simulink model "atrias_boom_nmSt_kinSw_v3"  (R2015a)
settings: Solver=ode23t  StartTime=0.0  StopTime=t_end  FixedStep=0.001  MaxStep=1e-3  RelTol=1e-3
InitFcn:
  | addpath('../common/')
  | colors
StartFcn:
  | tic
StopFcn:
  | %stopscript
values from neighbouring files (symbols this model uses):
  dt_a_dTrunk_boom = 5    [main_1_nmSt_kinSw.m]    (also in main_2_nmSt_kinSw_v2.m; main_3_nmSt_kinSw_v3.m; main_4_nmSt_kinSw_v4.m)
  dt_fade_boomCtrl = 2    [main_1_nmSt_kinSw.m]    (also in main_2_nmSt_kinSw_v2.m; main_3_nmSt_kinSw_v3.m; main_4_nmSt_kinSw_v4.m)
  initial_boom_yaw = 15*pi/180    (= 0.261799387799)    [main_2_nmSt_kinSw_v2.m]    (also in main_3_nmSt_kinSw_v3.m; main_4_nmSt_kinSw_v4.m)
  kd_boom_roll_Ctrl = 0    [main_1_nmSt_kinSw - Copy.m]    (also in main_1_nmSt_kinSw.m; main_2_nmSt_kinSw_v2.m; main_3_nmSt_kinSw_v3.m; main_4_nmSt_kinSw_v4.m)
  kd_boom_yaw_Ctrl = 0.1*kp_boom_yaw_Ctrl    (= 100000000)    [main_1_nmSt_kinSw - Copy.m]    (also in main_1_nmSt_kinSw.m = 1000000000; main_2_nmSt_kinSw_v2.m = 10000000; main_3_nmSt_kinSw_v3.m = 10000000; main_4_nmSt_kinSw_v4.m = 10000000)
  kd_motor = 0.90*2*sqrt(3.75*kp_motor)    [main_1_nmSt_kinSw - Copy.m]
  kinSw_alpha_start = 100*pi/180    (= 1.74532925199)    [main_1_nmSt_kinSw - Copy.m]    (also in main_1_nmSt_kinSw.m = 1.91986217719; main_2_nmSt_kinSw_v2.m = 1.83259571459; main_3_nmSt_kinSw_v3.m = 1.83259571459; main_4_nmSt_kinSw_v4.m = 1.83259571459)
  kinSw_alpha_tgt = 80*pi/180    (= 1.3962634016)    [main_1_nmSt_kinSw - Copy.m]    (also in main_1_nmSt_kinSw.m = 1.2217304764; main_2_nmSt_kinSw_v2.m = 1.2217304764; main_3_nmSt_kinSw_v3.m = 1.2217304764; main_4_nmSt_kinSw_v4.m = 1.2217304764)
  kinSw_t_start = 1.5    [main_1_nmSt_kinSw - Copy.m]    (also in main_1_nmSt_kinSw.m; main_2_nmSt_kinSw_v2.m = 0.5; main_3_nmSt_kinSw_v3.m = 0.5; main_4_nmSt_kinSw_v4.m = 0.5)
  kp_boom_roll_Ctrl = 0    [main_1_nmSt_kinSw - Copy.m]    (also in main_1_nmSt_kinSw.m; main_2_nmSt_kinSw_v2.m; main_3_nmSt_kinSw_v3.m; main_4_nmSt_kinSw_v4.m)
  kp_boom_yaw_Ctrl = 1e9    (= 1000000000)    [main_1_nmSt_kinSw - Copy.m]    (also in main_1_nmSt_kinSw.m = 10000000000; main_2_nmSt_kinSw_v2.m = 100000000; main_3_nmSt_kinSw_v3.m = 100000000; main_4_nmSt_kinSw_v4.m = 100000000)
  kp_motor = 3000    [main_1_nmSt_kinSw - Copy.m]
  max_back_bar_angle = 262.4*pi/180    (= 4.57974395723)    [main_1_nmSt_kinSw - Copy.m]
  max_front_bar_angle = 194.8*pi/180    (= 3.39990138288)    [main_1_nmSt_kinSw - Copy.m]
  min_back_bar_angle = 165.0*pi/180    (= 2.87979326579)    [main_1_nmSt_kinSw - Copy.m]
  min_front_bar_angle = 98.0*pi/180    (= 1.71042266695)    [main_1_nmSt_kinSw - Copy.m]
  poser_LLegAlp = (initial_l_leg_angle -pi/2)*180/pi    (= 105)    [main_2_nmSt_kinSw_v2.m]    (also in main_3_nmSt_kinSw_v3.m; main_4_nmSt_kinSw_v4.m)
  poser_LLegLen = initial_l_leg_length    (= 0.88)    [main_2_nmSt_kinSw_v2.m]    (also in main_3_nmSt_kinSw_v3.m; main_4_nmSt_kinSw_v4.m)
  poser_RLegAlp = (initial_r_leg_angle -pi/2)*180/pi    (= 75)    [main_2_nmSt_kinSw_v2.m]    (also in main_3_nmSt_kinSw_v3.m; main_4_nmSt_kinSw_v4.m)
  poser_RLegLen = initial_r_leg_length    (= 0.9)    [main_2_nmSt_kinSw_v2.m]    (also in main_3_nmSt_kinSw_v3.m; main_4_nmSt_kinSw_v4.m)
  tEnd_boomCtrl = t_end    (= 20)    [main_1_nmSt_kinSw - Copy.m]    (also in main_1_nmSt_kinSw.m = 3; main_2_nmSt_kinSw_v2.m = 7.5; main_3_nmSt_kinSw_v3.m = 7.5; main_4_nmSt_kinSw_v4.m = 7.5)
  tStart_boomCtrl = 1    [main_1_nmSt_kinSw - Copy.m]    (also in main_1_nmSt_kinSw.m = 0; main_2_nmSt_kinSw_v2.m = 0.5; main_3_nmSt_kinSw_v3.m = 0.5; main_4_nmSt_kinSw_v4.m = 0.5)
  tune_kinSw_alpha_start = kinSw_alpha_start*180/pi    (= 105)    [main_2_nmSt_kinSw_v2.m]    (also in main_3_nmSt_kinSw_v3.m; main_4_nmSt_kinSw_v4.m)
  tune_kinSw_alpha_tgt = kinSw_alpha_tgt*180/pi    (= 70)    [main_2_nmSt_kinSw_v2.m]    (also in main_3_nmSt_kinSw_v3.m; main_4_nmSt_kinSw_v4.m)
  tune_kinSw_len_min = kinSw_lclr    (= 0.7)    [main_2_nmSt_kinSw_v2.m]    (also in main_3_nmSt_kinSw_v3.m = 0.6)
  tune_kinSw_len_tgt = kinSw_len_tgt    (= 0.9)    [main_2_nmSt_kinSw_v2.m]    (also in main_3_nmSt_kinSw_v3.m)
  tune_M1_G = St_FGain_VAS*FmaxVAS    [main_2_nmSt_kinSw_v2.m]    (also in main_3_nmSt_kinSw_v3.m; main_4_nmSt_kinSw_v4.m)
  tune_M3_0 = CtrlPar_theta0*180/pi    [main_2_nmSt_kinSw_v2.m]    (also in main_3_nmSt_kinSw_v3.m; main_4_nmSt_kinSw_v4.m)
  tune_M3_D = St_GainDTh_HFL    [main_2_nmSt_kinSw_v2.m]    (also in main_3_nmSt_kinSw_v3.m; main_4_nmSt_kinSw_v4.m)
  tune_M3_P = St_GainTh_HFL    [main_2_nmSt_kinSw_v2.m]    (also in main_3_nmSt_kinSw_v3.m; main_4_nmSt_kinSw_v4.m)
  tune_M4_G = 1    [main_3_nmSt_kinSw_v3.m]    (also in main_4_nmSt_kinSw_v4.m)
  v_dTrunk_boom = 1.3    [main_1_nmSt_kinSw.m]    (also in main_2_nmSt_kinSw_v2.m; main_3_nmSt_kinSw_v3.m; main_4_nmSt_kinSw_v4.m)
undefined symbols (not defined in the file or in its folder): A1_notch_f1, A2_notch_f1, A_lpf_dtau, A_lpf_velocity, ankle_stiffness, B1_lpf_dtau, B1_lpf_velocity, B1_notch_f1, B2_lpf_dtau, B2_lpf_velocity, B2_notch_f1, b_hmotor, b_leg_spring, b_rotor, base_color_d, boom_color_d, boom_mount_to_center_diagonal, breakaway_friction, c_jointstop, contactThr, coulomb_friction, d_com, delta_phi_max, delta_phi_max_buffer, delta_phi_max_dropoff, delta_phi_min, fblink_color_d, floor_color_d, FmaxBFSH, FmaxGLU, FmaxHAM, FmaxHFL, FmaxRF, FmaxVAS, foot_color_d, FPCtrlPar, friction_linear_zone, g, gain_nodes_sea_torque, HIP_MTR_MAX_CONT_TORQUE, HIP_MTR_MAX_TORQUE, hshaft_color_d, initial_boom_pitch, initial_boom_roll, initial_hip_roll, initial_winch_angle, j_motor, k_gn, k_gt, k_leg_spring, K_notch_f1, k_phi, k_sea, Kb_leg, kd_lateral, kd_shin_max, kd_shin_min, kd_splay_max, kd_splay_min, kd_thigh_max ... (+186)
libraries: sm_lib x210, nesl_utility x140, simulink x65, simulink_extras x32, fl_lib x16, mblibv1 x2, commnoisgen2 x1
(part 7 of 17)

== system atrias_boom_nmSt_kinSw_v3/Mechanical System Layer/R Leg/Thigh ==
  CS1 to CS2 : sm_lib/Frames and Transforms/Rigid Transform  TranslationMethod=Cartesian  TranslationLengthUnit=m  TranslationStandardAxis=+Z  TranslationStandardOffset=0  TranslationCartesianOffset=[0 -l_seg 0]  TranslationROffset=0  TranslationROffsetUnits=m  TranslationZOffset=0  TranslationZOffsetUnits=m  TranslationThetaOffset=0  TranslationThetaOffsetUnits=deg  RotationMethod=None  RotationAngleUnits=deg  RotationStandardAxis=+Z  RotationAngle=0  RotationArbitraryAxis=[0 0 1]  FollAlignAxisA=+X  BaseAlignAxisA=+Y  FollAlignAxisB=+Y  BaseAlignAxisB=+Z  RotationMatrix=[1 0 0; 0 1 0; 0 0 1]  BlockFunction=simmechanics.library.frames_transforms.rigid_transform
  Frame Data : Subsystem
  Solid : sm_lib/Body Elements/Solid  InertiaType=Custom  Mass=m_thigh  MassUnits=kg  CenterOfMass=com_thigh  CenterOfMassUnits=m  MomentsOfInertia=i_thigh_moments  MomentsOfInertiaUnits=kg*m^2  ProductsOfInertia=i_thigh_products  ProductsOfInertiaUnits=kg*m^2  DensityBased=on  Density=1000  DensityUnits=kg/(m^3)  GraphicType=FromGeometry  MarkerShape=Sphere  MarkerSize=10  MarkerSizeUnits=m  GraphicVisPropType=AdvancedVisualProperties  GraphicDiffuseColor=thigh_color_d  GraphicSpecularColor=[0.5 0.5 0.5 1.0]  GraphicAmbientColor=[thigh_color_d*0.5 1.0]  GraphicEmissiveColor=[0.0 0.0 0.0 1.0]  GraphicShininess=128  GraphicOpacity=1.0  GeometryShape=FromFile  RectangleSize=[1 1]  RectangleSizeUnits=m  BrickDimensions=[1 1 1]  BrickDimensionUnits=m  CylinderRadius=l_rad  CylinderRadiusUnits=m  CylinderLength=l_seg  CylinderLengthUnits=m  SphereRadius=1  SphereRadiusUnits=m  EllipsoidRadii=[1 1 1]  EllipsoidRadiiUnits=m  ExtrusionCrossSection=[1 1; -1 1; -1 -1; 1 -1]  ExtrusionCrossSectionUnits=m  ExtrusionLength=1  ExtrusionLengthUnits=m  PolygonNumSides=3  PolygonOuterRadius=1  PolygonOuterRadiusUnits=m  ExtGeomFileType=STL  ExtGeomFileName=../models/thigh.STL  ExtGeomFileUnits=m  RevolutionCrossSection=[1 1; 1 -1; 2 -1; 2 1]  RevolutionCrossSectionUnits=m  RevolutionExtent=Full  RevolutionAngle=180  RevolutionAngleUnits=deg  BlockFunction=simmechanics.library.body_elements.solid
  CS1 : PMIOPort  Port=1  Side=Left
  CS2 : PMIOPort  Port=2  Side=Right
  connections:
  CS2/RConn1 -- CS1 to CS2/RConn1
  CS1 to CS2/LConn1 -- Solid/RConn1 -- Frame Data/LConn1 -- CS1/RConn1

== system atrias_boom_nmSt_kinSw_v3/Mechanical System Layer/R Leg/Thigh SEA ==
  note: Thigh SEA Mechanics
  Thigh Gear Torque [Nm] : Inport
  Thigh Joint [rad rad/s] : Inport  Port=2
  Continuous Angle : mblibv1/Utilities/Continuous Angle  rad=rad  rads=rad/s
  Demux : Demux  Outputs=2
  Gain : Gain  Gain=k_leg_spring
  Gain1 : Gain  Gain=b_leg_spring
  Initial Gear Angle : Constant  Value=thigh_initial_r
  Inverse Gear Ratio1 : Gain  Gain=1/N
  Inverse Gear Ratio2 : Gain  Gain=Kt_leg
  Inverse Gear Ratio3 : Gain  Gain=1/Kt_leg
  Motor Efficiency : Gain  Gain=mu_motor
  Motor Controller : Subsystem  Commented=on
  Motor Electromagnetism : Subsystem  Commented=on
  Rotor Damping : Gain  Gain=b_rotor
  Rotor and Gearing : Subsystem
  Sum : Sum  Inputs=++|
  Sum2 : Sum  Inputs=+|-
  Sum3 : Sum  Inputs=|+-
  Sum4 : Sum  Inputs=+|-
  Sum5 : Sum  Inputs=|++
  Torque Limiter (outside) 2 : Saturate  UpperLimit=LEG_MTR_MAX_TORQUE  LowerLimit=-LEG_MTR_MAX_TORQUE  ZeroCross=off
      settings: AttributesFormatString=Hi: %<UpperLimit>\nLo: %<LowerLimit>
  Rotor Joint Conn : PMIOPort  Port=1  Side=Left
  Thigh Joint Torque [Nm] : Outport
  Thigh Gear [rad] : Outport  Port=2
  wires:
  Sum2/1 -> Gain/1
  Sum3/1 -> Motor Efficiency/1
  Rotor Damping/1 -> Sum3/2
  Gain/1 -> Sum5/1  "tau_load"
  Gain1/1 -> Sum5/2
  Sum4/1 -> Gain1/1
  Thigh Joint [rad rad/s]/1 -> Demux/1
  Demux/1 -> Sum2/2
  Demux/2 -> Sum4/2
  Inverse Gear Ratio3/1 -> Inverse Gear Ratio2/1
  Inverse Gear Ratio2/1 -> Sum3/1
  Initial Gear Angle/1 -> Sum/1
  Sum/1 -> Thigh Gear [rad]/1, Sum2/1
  Continuous Angle/1 -> Sum/2
  Rotor and Gearing/1(Gearhead Position [rad]) -> Continuous Angle/1
  Motor Controller/1(Voltage [V]) -> Motor Electromagnetism/1(Voltage [V])
  Motor Electromagnetism/1(Current [A]) -> Motor Controller/2(Measured Current [A])
  Thigh Gear Torque [Nm]/1 -> Torque Limiter (outside) 2/1
  Inverse Gear Ratio1/1 -> Inverse Gear Ratio3/1
  Motor Efficiency/1 -> Rotor and Gearing/1(Rotor Torque [Nm])
  Rotor and Gearing/2(Gearhead Velocity [rad/s]) -> Sum4/1, Continuous Angle/2
  Sum5/1 -> Thigh Joint Torque [Nm]/1, Rotor and Gearing/2(Spring Torque [Nm])
  Rotor and Gearing/3(Rotor Velocity [rad/s]) -> Rotor Damping/1
  Torque Limiter (outside) 2/1 -> Inverse Gear Ratio1/1
  connections:
  Rotor and Gearing/LConn1 -- Rotor Joint Conn/RConn1

== system atrias_boom_nmSt_kinSw_v3/Mechanical System Layer/Right Hip Roll Joint/Mechanical Limits  ==
  vphi : Inport
  phi : Inport  Port=2
  Compare To Constant5 : simulink/Logic and Bit Operations/Compare To Constant  relop=<=  const=phi_max_collision  OutDataTypeStr=boolean  ZeroCross=off
  Compare To Zero1 : simulink/Logic and Bit Operations/Compare To Zero  relop=<=  OutDataTypeStr=boolean  ZeroCross=off
  Compare To Zero2 : simulink/Logic and Bit Operations/Compare To Zero  relop=<=  OutDataTypeStr=boolean  ZeroCross=off
  Constant1 : Constant  Value=phi_roll_min
  Constant2 : Constant  Value=phi_roll_max
  Enabled Subsystem : Subsystem  TreatAsAtomicUnit=on
  Gain2 : Gain  Gain=-1
  Logical Operator : Logic  Operator=OR  Inputs=1  AllPortsSameDT=off  OutDataTypeStr=boolean
  Mux : Mux  Inputs=2
  Roll Max Collision Model : Subsystem
  Roll Min Collision Model : Subsystem
  Stop Simulation6 : Stop
  Sum1 : Sum  Inputs=-+|
  Sum11 : Sum  Inputs=-|+
  Sum5 : Sum  Inputs=+-|
  tau_reaction : Outport
  wires:
  Sum1/1 -> [col_hip_min], Compare To Zero1/1, Roll Min Collision Model/1(phi [rad])
  Roll Min Collision Model/1(tau_interaction[Nm]) -> Sum11/2
  Compare To Zero1/1 -> Roll Min Collision Model/Enable
  phi/1 -> Sum1/2, Sum5/2
  Logical Operator/1 -> Stop Simulation6/1, Enabled Subsystem/Enable
  [col_hip_max] -> Mux/1
  Mux/1 -> Compare To Constant5/1
  [col_hip_min] -> Mux/2
  Sum11/1 -> tau_reaction/1
  Constant1/1 -> Sum1/1
  Compare To Constant5/1 -> Enabled Subsystem/1(Col_Flags), Logical Operator/1
  Constant2/1 -> Sum5/1
  Sum5/1 -> [col_hip_max], Compare To Zero2/1, Roll Max Collision Model/1(phi [rad])
  Compare To Zero2/1 -> Roll Max Collision Model/Enable
  Roll Max Collision Model/1(tau_interaction[Nm]) -> Sum11/1
  vphi/1 -> Roll Min Collision Model/2(vphi [rad/s]), Gain2/1
  Gain2/1 -> Roll Max Collision Model/2(vphi [rad/s])

== system atrias_boom_nmSt_kinSw_v3/Mechanical System Layer/Torso/COM Sensor ==
  Mux : Mux  Inputs=3
  PS-Simulink Converter{1,3..8} (7 alike) : nesl_utility/PS-Simulink Converter  PhysicalDomain=network_engine_domain  SubClassName=ps_output  LeftPortType=input  RightPortType=output  PseudoPeriodic=off  Frequencies=[]  Unit=1  AffineConversion=off
  Transform Sensor : sm_lib/Frames and Transforms/Transform Sensor  MeasurementFrame=World  SenseAngle=off  SenseAxis=off  SenseAngle1=off  SenseAngle2=off  SenseAngle3=off  SenseQ=off  SenseR=off  SenseOmegaX=off  SenseOmegaY=off  SenseOmegaZ=off  SenseOmega1=off  SenseOmega2=off  SenseOmega3=off  SenseQDot=off  SenseRDot=off  SenseAlphaX=off  SenseAlphaY=off  SenseAlphaZ=off  SenseAlpha1=off  SenseAlpha2=off  SenseAlpha3=off  SenseQDDot=off  SenseRDDot=off  SenseX=off  SenseY=on  SenseZ=off  SenseRad=off  SenseAzim=off  SenseDist=off  SenseInc=off  SenseXDot=on  SenseYDot=on  SenseZDot=on  SenseRadDot=off  SenseAzimDot=off  SenseDistDot=off  SenseIncDot=off  SenseXDDot=on  SenseYDDot=on  SenseZDDot=on  SenseRadDDot=off  SenseAzimDDot=off  SenseDistDDot=off  SenseIncDDot=off  BlockFunction=simmechanics.library.frames_transforms.transform_sensor
  Transverse Component : Subsystem
  World Frame : sm_lib/Frames and Transforms/World Frame  BlockFunction=simmechanics.library.frames_transforms.world_frame
  COM : PMIOPort  Port=1  Side=Left
  Acceleration : Outport
  y : Outport  Port=2
  dx : Outport  Port=3
  dy : Outport  Port=4
  wires:
  PS-Simulink Converter5/1 -> Mux/3
  Mux/1 -> Acceleration/1
  PS-Simulink Converter8/1 -> y/1
  PS-Simulink Converter3/1 -> Mux/2
  PS-Simulink Converter4/1 -> Mux/1
  PS-Simulink Converter7/1 -> Transverse Component/1(x)
  Transverse Component/1(transverse) -> dx/1
  [qYaw] -> Transverse Component/3(yaw)
  PS-Simulink Converter1/1 -> dy/1
  PS-Simulink Converter6/1 -> Transverse Component/2(z)
  connections:
  COM/RConn1 -- Transform Sensor/RConn1
  World Frame/RConn1 -- Transform Sensor/LConn1
  PS-Simulink Converter5/LConn1 -- Transform Sensor/RConn8
  PS-Simulink Converter3/LConn1 -- Transform Sensor/RConn7
  PS-Simulink Converter4/LConn1 -- Transform Sensor/RConn6
  PS-Simulink Converter6/LConn1 -- Transform Sensor/RConn5
  PS-Simulink Converter7/LConn1 -- Transform Sensor/RConn3
  PS-Simulink Converter8/LConn1 -- Transform Sensor/RConn2
  PS-Simulink Converter1/LConn1 -- Transform Sensor/RConn4

== system atrias_boom_nmSt_kinSw_v3/Mechanical System Layer/Torso/Frame Data ==
  Kinematic Data : ToWorkspace  VariableName=torso_out  SampleTime=output_sample_time
      settings: Save2DSignal=2-D array (concatenate along first dimension)
  Mux : Mux
  PS-Simulink Converter{,1..3} (4 alike) : nesl_utility/PS-Simulink Converter  PhysicalDomain=network_engine_domain  SubClassName=ps_output  LeftPortType=input  RightPortType=output  PseudoPeriodic=off  Frequencies=[]  Unit=1  AffineConversion=off
  Transform Sensor : sm_lib/Frames and Transforms/Transform Sensor  MeasurementFrame=World  SenseAngle=off  SenseAxis=off  SenseAngle1=off  SenseAngle2=off  SenseAngle3=off  SenseQ=on  SenseR=off  SenseOmegaX=off  SenseOmegaY=off  SenseOmegaZ=off  SenseOmega1=off  SenseOmega2=off  SenseOmega3=off  SenseQDot=off  SenseRDot=off  SenseAlphaX=off  SenseAlphaY=off  SenseAlphaZ=off  SenseAlpha1=off  SenseAlpha2=off  SenseAlpha3=off  SenseQDDot=off  SenseRDDot=off  SenseX=on  SenseY=on  SenseZ=on  SenseRad=off  SenseAzim=off  SenseDist=off  SenseInc=off  SenseXDot=off  SenseYDot=off  SenseZDot=off  SenseRadDot=off  SenseAzimDot=off  SenseDistDot=off  SenseIncDot=off  SenseXDDot=off  SenseYDDot=off  SenseZDDot=off  SenseRadDDot=off  SenseAzimDDot=off  SenseDistDDot=off  SenseIncDDot=off  BlockFunction=simmechanics.library.frames_transforms.transform_sensor
  World Frame : sm_lib/Frames and Transforms/World Frame  BlockFunction=simmechanics.library.frames_transforms.world_frame
  Frame : PMIOPort  Port=1  Side=Left
  wires:
  Mux/1 -> Kinematic Data/1
  PS-Simulink Converter/1 -> Mux/1
  PS-Simulink Converter1/1 -> Mux/2
  PS-Simulink Converter2/1 -> Mux/3
  PS-Simulink Converter3/1 -> Mux/4
  connections:
  PS-Simulink Converter3/LConn1 -- Transform Sensor/RConn5
  PS-Simulink Converter2/LConn1 -- Transform Sensor/RConn4
  PS-Simulink Converter1/LConn1 -- Transform Sensor/RConn3
  PS-Simulink Converter/LConn1 -- Transform Sensor/RConn2
  Transform Sensor/RConn1 -- Frame/RConn1
  Transform Sensor/LConn1 -- World Frame/RConn1

== system atrias_boom_nmSt_kinSw_v3/Mechanical System Layer/Yaw Shaft/Frame Data ==
  Kinematic Data : ToWorkspace  VariableName=boom_yaw_out  SampleTime=output_sample_time
      settings: Save2DSignal=2-D array (concatenate along first dimension)
  Mux : Mux
  PS-Simulink Converter{,1..3} (4 alike) : nesl_utility/PS-Simulink Converter  PhysicalDomain=network_engine_domain  SubClassName=ps_output  LeftPortType=input  RightPortType=output  PseudoPeriodic=off  Frequencies=[]  Unit=1  AffineConversion=off
  Transform Sensor : sm_lib/Frames and Transforms/Transform Sensor  MeasurementFrame=World  SenseAngle=off  SenseAxis=off  SenseAngle1=off  SenseAngle2=off  SenseAngle3=off  SenseQ=on  SenseR=off  SenseOmegaX=off  SenseOmegaY=off  SenseOmegaZ=off  SenseOmega1=off  SenseOmega2=off  SenseOmega3=off  SenseQDot=off  SenseRDot=off  SenseAlphaX=off  SenseAlphaY=off  SenseAlphaZ=off  SenseAlpha1=off  SenseAlpha2=off  SenseAlpha3=off  SenseQDDot=off  SenseRDDot=off  SenseX=on  SenseY=on  SenseZ=on  SenseRad=off  SenseAzim=off  SenseDist=off  SenseInc=off  SenseXDot=off  SenseYDot=off  SenseZDot=off  SenseRadDot=off  SenseAzimDot=off  SenseDistDot=off  SenseIncDot=off  SenseXDDot=off  SenseYDDot=off  SenseZDDot=off  SenseRadDDot=off  SenseAzimDDot=off  SenseDistDDot=off  SenseIncDDot=off  BlockFunction=simmechanics.library.frames_transforms.transform_sensor
  World Frame : sm_lib/Frames and Transforms/World Frame  BlockFunction=simmechanics.library.frames_transforms.world_frame
  Frame : PMIOPort  Port=1  Side=Left
  wires:
  Mux/1 -> Kinematic Data/1
  PS-Simulink Converter/1 -> Mux/1
  PS-Simulink Converter1/1 -> Mux/2
  PS-Simulink Converter2/1 -> Mux/3
  PS-Simulink Converter3/1 -> Mux/4
  connections:
  PS-Simulink Converter3/LConn1 -- Transform Sensor/RConn5
  PS-Simulink Converter2/LConn1 -- Transform Sensor/RConn4
  PS-Simulink Converter1/LConn1 -- Transform Sensor/RConn3
  PS-Simulink Converter/LConn1 -- Transform Sensor/RConn2
  Transform Sensor/RConn1 -- Frame/RConn1
  Transform Sensor/LConn1 -- World Frame/RConn1

== system atrias_boom_nmSt_kinSw_v3/Control/Actuator Control/SEA Controller (Torque)/Antiresonance Compensation ==
  Torque : Inport
  Notch Filter (Flight) : DiscreteTransferFcn  Numerator=[K_notch_f1 K_notch_f1*A1_notch_f1 K_notch_f1*A2_notch_f1]  Denominator=[1 B1_notch_f1 B2_notch_f1]  SampleTime=sample_time
  Filtered Torque : Outport
  wires:
  Notch Filter (Flight)/1 -> Filtered Torque/1
  Torque/1 -> Notch Filter (Flight)/1

== system atrias_boom_nmSt_kinSw_v3/Control/Actuator Control/SEA Controller (Torque)/Friction Compensation ==
  Motor Velocity [rad/s] : Inport
  Gain2 : Gain  Gain=sea_coulomb_friction_direction_switch_sensitivity
  KdGain2 : Gain  Description=xPCTag(1)=kd_sea_torque;  Gain=sea_coulomb_friction
  Trigonometric Function : Trigonometry  Operator=tanh
  Friction Compensation [Nm] : Outport
  wires:
  Trigonometric Function/1 -> KdGain2/1
  Gain2/1 -> Trigonometric Function/1
  Motor Velocity [rad/s]/1 -> Gain2/1
  KdGain2/1 -> Friction Compensation [Nm]/1

== system atrias_boom_nmSt_kinSw_v3/Control/Actuator Control/SEA Controller (Torque)/Loaded Unloaded Switch ==
  Loaded Signal : Inport
  Unloaded Signal : Inport  Port=2
  Loaded/Unloaded [1/0] x4 : Inport  Port=3
  Demux : Demux
  Demux1 : Demux
  Demux2 : Demux
  Mux : Mux
  Switch{,1..3} (4 alike) : Switch  Criteria=u2 ~= 0
  Signal : Outport
  wires:
  Demux2/1 -> Switch/3
  Demux2/2 -> Switch1/3
  Demux2/3 -> Switch2/3
  Demux2/4 -> Switch3/3
  Unloaded Signal/1 -> Demux2/1
  Demux1/4 -> Switch3/1
  Demux1/3 -> Switch2/1
  Demux1/2 -> Switch1/1
  Demux1/1 -> Switch/1
  Loaded Signal/1 -> Demux1/1
  Demux/1 -> Switch/2
  Switch/1 -> Mux/1
  Mux/1 -> Signal/1
  Loaded/Unloaded [1/0] x4/1 -> Demux/1
  Switch3/1 -> Mux/4
  Switch2/1 -> Mux/3
  Switch1/1 -> Mux/2
  Demux/2 -> Switch1/2
  Demux/3 -> Switch2/2
  Demux/4 -> Switch3/2

== system atrias_boom_nmSt_kinSw_v3/Control/Actuator Control/SEA Controller (Torque)/critical damping ==
  p gain : Inport
  Gain : Gain  Gain=1.0
  Gain1 : Gain  Gain=2
  Gain2 : Gain  Gain=j_motor
  Spring Stiffness1 : Gain  Gain=1./k_sea
  Sqrt : Sqrt  SaturateOnIntegerOverflow=on
  d gain : Outport
  wires:
  p gain/1 -> Spring Stiffness1/1
  Gain/1 -> Gain1/1
  Sqrt/1 -> Gain/1
  Gain2/1 -> Sqrt/1
  Spring Stiffness1/1 -> Gain2/1
  Gain1/1 -> d gain/1

== system atrias_boom_nmSt_kinSw_v3/Control/Behavior Control/Add Limit Avoidance PD Torques/mechanical limit avoidance ==
  tau_des [Nm]x4 : Inport
  PD Joint Limit : Subsystem
  Product : Product
  Sum : Sum  Inputs=++|
  tau_des + pd [Nm]x4 : Outport
  wires:
  tau_des [Nm]x4/1 -> Product/2
  PD Joint Limit/1(tau_pd [Nm]x4) -> Sum/1
  Sum/1 -> tau_des + pd [Nm]x4/1
  PD Joint Limit/2(des_trq_scale x4) -> Product/1
  Product/1 -> Sum/2

== system atrias_boom_nmSt_kinSw_v3/Control/Behavior Control/Robot-to-NMM Interface/L Leg Load ==
  tau_F [Nm] : Inport
  tau_B [Nm] : Inport  Port=2
  splay [rad] : Inport  Port=3
  Calculate Leg Load : Fcn  Expr=1/(2*l_seg*sin(u(3)/2))*u(1)-1/(2*l_seg*sin(u(3)/2))*u(2)
  Calculate Tangential Leg Force : Fcn  Expr=1/(2*l_seg*cos(u(3)/2))*(u(1)+u(2))
  Mux : Mux  Inputs=3
  Positive Values only : Saturate  UpperLimit=Inf  LowerLimit=0
  Leg Load [N] : Outport
  F_t (tangential leg force) [N] : Outport  Port=2
  wires:
  Calculate Leg Load/1 -> Positive Values only/1
  Positive Values only/1 -> Leg Load [N]/1
  Mux/1 -> Calculate Tangential Leg Force/1, Calculate Leg Load/1
  splay [rad]/1 -> Mux/3
  tau_B [Nm]/1 -> Mux/2
  tau_F [Nm]/1 -> Mux/1
  Calculate Tangential Leg Force/1 -> F_t (tangential leg force) [N]/1

== system atrias_boom_nmSt_kinSw_v3/Control/Behavior Control/Robot-to-NMM Interface/R GRF ==
  F_l [N] : Inport
  F_t [N] : Inport  Port=2
  alpha [rad] : Inport  Port=3
  Constant : Constant
  GRF tangential (x) : Fcn  Expr=-u(1)*cos(u(3)) + u(2)*sin(u(3))
  GRF vertical : Fcn  Expr=u(1)*sin(u(3)) + u(2)*cos(u(3))
  Mux : Mux  Inputs=3
  Mux1 : Mux  Inputs=3
  GRF_xyz [N N N] : Outport
  wires:
  alpha [rad]/1 -> Mux/3
  F_t [N]/1 -> Mux/2
  F_l [N]/1 -> Mux/1
  Mux/1 -> GRF tangential (x)/1, GRF vertical/1
  GRF tangential (x)/1 -> Mux1/1
  GRF vertical/1 -> Mux1/2

== system atrias_boom_nmSt_kinSw_v3/Control/Behavior Control/Robot-to-NMM Interface/R Leg Geometry f(l_seg, l_v, v12_max) ==
  qBack [rad] : Inport
  qFront [rad] : Inport  Port=2
  dqBack [rad/s] : Inport  Port=3
  dqFront [rad/s] : Inport  Port=4
  Constant : Constant  Value=pi/2
  Constant1 : Constant  Value=l_seg/l_v
  Divide : Product  Inputs=**/
  Fcn : Fcn  Expr=(1-u(3))/2*u(1) + (1+u(3))/2*u(2)
  Fcn1 : Fcn  Expr=-u(3)*u(1) + u(3)*u(2)
  Gain : Gain  Gain=0.5
  Gain1 : Gain  Gain=0.5
  Gain2 : Gain  Gain=l_seg/l_v
  Gain3 : Gain  Gain=2
  Gain4 : Gain  Gain=0.5
  Mux : Mux  Inputs=3
  Sum : Sum  Inputs=|+-
  Sum1 : Sum  Inputs=|+-
  Sum2 : Sum  Inputs=|++
  Sum3 : Sum  Inputs=|++
  Trigonometric Function : Trigonometry  Operator=cos
  Trigonometric Function1 : Trigonometry  Operator=asin
  Trigonometric Function2 : Trigonometry
  Trigonometric Function3 : Trigonometry  Operator=cos
  "[0,sin(v12_max/2)]" : Saturate  UpperLimit=sin(v12_max/2)  LowerLimit=0
  "[0,v12_max]" : Saturate  UpperLimit=v12_max  LowerLimit=0
  "[min_splay_angle/2, inf]" : Saturate  UpperLimit=inf  LowerLimit=min_splay_angle/2
  virtual knee angle [rad] : Outport
  virtual knee velocity [rad/s] : Outport  Port=2
  virtual hip angle [rad] : Outport  Port=3
  virtual hip velocity [rad/s] : Outport  Port=4
  k : Outport  Port=5
  wires:
  Sum/1 -> Gain/1
  qBack [rad]/1 -> [qB]
  qFront [rad]/1 -> [qF]
  dqBack [rad/s]/1 -> [dqB]
  dqFront [rad/s]/1 -> [dqF]
  [qF] -> Sum3/2, Sum/2
  [qB] -> Sum/1, Sum3/1
  Gain/1 -> Trigonometric Function/1, "[min_splay_angle/2, inf]"/1
  [phiK] -> Gain1/1
  Sum1/1 -> Sum2/1
  Constant/1 -> Sum1/2
  Gain1/1 -> Trigonometric Function3/1, Sum2/2
  Sum2/1 -> [phiH]
  Trigonometric Function/1 -> Gain2/1
  Gain2/1 -> "[0,sin(v12_max/2)]"/1
  "[0,sin(v12_max/2)]"/1 -> Trigonometric Function1/1
  Trigonometric Function1/1 -> "[0,v12_max]"/1
  "[0,v12_max]"/1 -> Gain3/1
  Gain3/1 -> [phiK]
  [phiK] -> virtual knee angle [rad]/1
  [phiH] -> virtual hip angle [rad]/1
  Trigonometric Function2/1 -> Divide/2
  Constant1/1 -> Divide/1
  Trigonometric Function3/1 -> Divide/3
  Divide/1 -> k/1, Mux/3
  Mux/1 -> Fcn/1, Fcn1/1
  [dqF] -> Mux/2
  [dqB] -> Mux/1
  Fcn/1 -> virtual hip velocity [rad/s]/1
  Fcn1/1 -> virtual knee velocity [rad/s]/1
  Sum3/1 -> Gain4/1
  Gain4/1 -> Sum1/1
  "[min_splay_angle/2, inf]"/1 -> Trigonometric Function2/1

== system atrias_boom_nmSt_kinSw_v3/Control/Behavior Control/Robot-to-NMM Interface/R Leg Geometry f(l_seg, l_v, v12_max)1 ==
  qBack [rad] : Inport
  qFront [rad] : Inport  Port=2
  dqBack [rad/s] : Inport  Port=3
  dqFront [rad/s] : Inport  Port=4
  Constant : Constant  Value=pi/2
  Constant1 : Constant  Value=l_seg/l_v
  Divide : Product  Inputs=**/
  Fcn : Fcn  Expr=(1-u(3))/2*u(1) + (1+u(3))/2*u(2)
  Fcn1 : Fcn  Expr=-u(3)*u(1) + u(3)*u(2)
  Gain : Gain  Gain=0.5
  Gain1 : Gain  Gain=0.5
  Gain2 : Gain  Gain=l_seg/l_v
  Gain3 : Gain  Gain=2
  Gain4 : Gain  Gain=0.5
  Mux : Mux  Inputs=3
  Sum : Sum  Inputs=|+-
  Sum1 : Sum  Inputs=|+-
  Sum2 : Sum  Inputs=|++
  Sum3 : Sum  Inputs=|++
  Trigonometric Function : Trigonometry  Operator=cos
  Trigonometric Function1 : Trigonometry  Operator=asin
  Trigonometric Function2 : Trigonometry
  Trigonometric Function3 : Trigonometry  Operator=cos
  "[0,sin(v12_max/2)]" : Saturate  UpperLimit=sin(v12_max/2)  LowerLimit=0
  "[0,v12_max]" : Saturate  UpperLimit=v12_max  LowerLimit=0
  "[min_splay_angle/2, inf]" : Saturate  UpperLimit=inf  LowerLimit=min_splay_angle/2
  virtual knee angle [rad] : Outport
  virtual knee velocity [rad/s] : Outport  Port=2
  virtual hip angle [rad] : Outport  Port=3
  virtual hip velocity [rad/s] : Outport  Port=4
  k : Outport  Port=5
  wires:
  "[min_splay_angle/2, inf]"/1 -> Trigonometric Function2/1
  Gain4/1 -> Sum1/1
  Sum3/1 -> Gain4/1
  Fcn1/1 -> virtual knee velocity [rad/s]/1
  Fcn/1 -> virtual hip velocity [rad/s]/1
  [dqB] -> Mux/1
  [dqF] -> Mux/2
  Mux/1 -> Fcn1/1, Fcn/1
  Divide/1 -> Mux/3, k/1
  Trigonometric Function3/1 -> Divide/3
  Constant1/1 -> Divide/1
  Trigonometric Function2/1 -> Divide/2
  [phiH] -> virtual hip angle [rad]/1
  [phiK] -> virtual knee angle [rad]/1
  Gain3/1 -> [phiK]
  "[0,v12_max]"/1 -> Gain3/1
  Trigonometric Function1/1 -> "[0,v12_max]"/1
  "[0,sin(v12_max/2)]"/1 -> Trigonometric Function1/1
  Gain2/1 -> "[0,sin(v12_max/2)]"/1
  Trigonometric Function/1 -> Gain2/1
  Sum2/1 -> [phiH]
  Gain1/1 -> Sum2/2, Trigonometric Function3/1
  Constant/1 -> Sum1/2
  Sum1/1 -> Sum2/1
  [phiK] -> Gain1/1
  Gain/1 -> "[min_splay_angle/2, inf]"/1, Trigonometric Function/1
  [qB] -> Sum3/1, Sum/1
  [qF] -> Sum/2, Sum3/2
  dqFront [rad/s]/1 -> [dqF]
  dqBack [rad/s]/1 -> [dqB]
  qFront [rad]/1 -> [qF]
  qBack [rad]/1 -> [qB]
  Sum/1 -> Gain/1

== system atrias_boom_nmSt_kinSw_v3/Control/Behavior Control/Robot-to-NMM Interface/R Leg Load ==
  tau_F [Nm] : Inport
  tau_B [Nm] : Inport  Port=2
  splay [rad] : Inport  Port=3
  Calculate Leg Load : Fcn  Expr=1/(2*l_seg*sin(u(3)/2))*u(1)-1/(2*l_seg*sin(u(3)/2))*u(2)
  Calculate Tangential Leg Force : Fcn  Expr=1/(2*l_seg*cos(u(3)/2))*(u(1)+u(2))
  Mux : Mux  Inputs=3
  Positive Values only : Saturate  UpperLimit=Inf  LowerLimit=0
  Leg Load [N] : Outport
  F_t (tangential leg force) [N] : Outport  Port=2
  wires:
  Calculate Leg Load/1 -> Positive Values only/1
  Positive Values only/1 -> Leg Load [N]/1
  Mux/1 -> Calculate Tangential Leg Force/1, Calculate Leg Load/1
  splay [rad]/1 -> Mux/3
  tau_B [Nm]/1 -> Mux/2
  tau_F [Nm]/1 -> Mux/1
  Calculate Tangential Leg Force/1 -> F_t (tangential leg force) [N]/1

== system atrias_boom_nmSt_kinSw_v3/Control/Behavior Control/Virtual Neuromuscular Control/Higher Control Layer ==
  note: Target Foot Placement
  note: Target Swing Leg Length
      | (constant)
  note: Stance to Swing Leg Decision
  note: Target Trunk Angle
      | (constant)
  note: Higher Control Layer
      | (Supra Spinal Control)
  Double Support : Subsystem
  Mux{1..4} (4 alike) : Mux  Inputs=2
  Sum{1..4} (4 alike) : Sum  Inputs=-+|
  left alpha_tgt (sagittal) : Fcn  Expr=u(1) + u(2)*u(4) + u(3)*u(5)
  right alpha_tgt (sagittal) : Fcn  Expr=u(1) + u(2)*u(4) + u(3)*u(5)
  tag scope: Lalpha_tgt=global, LonR=global, Ralpha_tgt=global, RonL=global, double_support=global, flight=global, flight_LonR=global, flight_RonL=global, leg_clr=global, theta_tgt=global
  wires:
  left alpha_tgt (sagittal)/1 -> [Lalpha_tgt]
  right alpha_tgt (sagittal)/1 -> [Ralpha_tgt]
  [LLCtrlPar] -> [leg_clr]
  Double Support/3(LonR) -> [LonR]
  [LStance] -> Double Support/1(LStance)
  [RStance] -> Double Support/2(RStance)
  Double Support/1(RonL) -> [RonL]
  Double Support/2(Flight) -> [flight]
  Sum1/1 -> Double Support/3(Lalpha_tgt)
  [Lphi23] -> Double Support/4(Lphi34)
  [Rphi23] -> Double Support/7(Rphi34)
  [Lphi12] -> Double Support/5(Lphi23)
  [Rphi12] -> Double Support/8(Rphi23)
  [Lalpha_tgt] -> Sum1/2
  [theta] -> Sum1/1, Sum2/1
  [Ralpha_tgt] -> Sum2/2
  [theta0] -> [theta_tgt]
  Mux1/1 -> left alpha_tgt (sagittal)/1
  [FPCtrlPar] -> Mux4/1, Mux1/1
  Mux2/1 -> Mux1/2
  Mux4/1 -> right alpha_tgt (sagittal)/1
  Mux3/1 -> Mux4/2
  [xRShank1] -> Sum3/1
  [xTorso] -> Sum3/2, Sum4/2
  Sum3/1 -> Mux2/1
  [xLShank1] -> Sum4/1
  Sum4/1 -> Mux3/1
  [dxTorso] -> Mux3/2, Mux2/2
  Double Support/4(DS) -> [double_support]
  Sum2/1 -> Double Support/6(Ralpha_tgt)
  Double Support/5(RonL (Flight)) -> [flight_RonL]
  Double Support/6(LonR (Flight)) -> [flight_LonR]

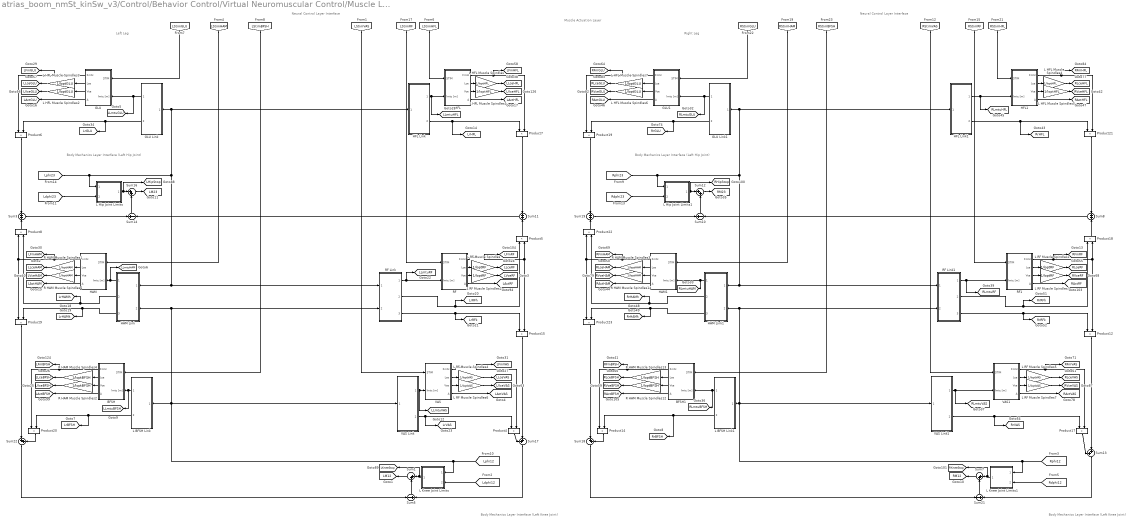
== system atrias_boom_nmSt_kinSw_v3/Control/Behavior Control/Virtual Neuromuscular Control/Muscle Layer ==
  note: Left Leg
  note: Neural Control Layer Interface
  note: Muscle Actuation Layer
  note: Body Mechanics Layer
      | Interface (Left Hip Joint)
  note: Body Mechanics Layer
      | Interface (Left Knee Joint)
  note: Right Leg
  note: Neural Control Layer Interface
  note: Body Mechanics Layer
      | Interface (Left Hip Joint)
  note: Body Mechanics Layer
      | Interface (Left Knee Joint)
  BFSH : Subsystem
  BFSH1 : Subsystem
  GLU : Subsystem
  GLU Link : Subsystem
  GLU Link1 : Subsystem
  GLU1 : Subsystem
  HAM : Subsystem
  HAM Link : Subsystem
  HAM Link1 : Subsystem
  HAM1 : Subsystem
  HFL : Subsystem
  HFL Link : Subsystem
  HFL Link1 : Subsystem
  HFL1 : Subsystem
  L BFSH Link : Subsystem
  L BFSH Link1 : Subsystem
  L HFL Muscle Spindles{,1,4..5} (4 alike) : Gain  Gain=1/loptHFL
  L HFL Muscle Spindles{2..3,6..7} (4 alike) : Gain  Gain=1/loptGLU
  L Hip Joint Limits : Subsystem
  L Hip Joint Limits1 : Subsystem
  L Knee Joint Limits : Subsystem
  L Knee Joint Limits1 : Subsystem
  L RF Muscle Spindles{,1..3} (4 alike) : Gain  Gain=1/loptRF
  L RF Muscle Spindles{4..7} (4 alike) : Gain  Gain=1/loptVAS
  Product{4..9,12,14..15,17..23} (16 alike) : Product  RndMeth=Zero
  R HAM Muscle Spindles{1,3,6,14} (4 alike) : Gain  Gain=1/loptHAM
  R HAM Muscle Spindles{2,4,12..13} (4 alike) : Gain  Gain=1/loptBFSH
  RF : Subsystem
  RF Link : Subsystem
  RF Link1 : Subsystem
  RF1 : Subsystem
  Sum{1,7,12,16,18,22} (6 alike) : Sum  Inputs=|++
  Sum10 : Sum  Inputs=+-
  Sum{3,8,11,19} (4 alike) : Sum
  Sum13 : Sum  Inputs=++|
  Sum14 : Sum  Inputs=+-
  Sum17 : Sum  Inputs=++|
  Sum21 : Sum  Inputs=-+
  Sum5 : Sum  Inputs=-+
  VAS : Subsystem
  VAS Link : Subsystem
  VAS Link1 : Subsystem
  VAS1 : Subsystem
  tag scope: LActBFSH=global, LActGLU=global, LActHAM=global, LActHFL=global, LActRF=global, LActVAS=global, LFmBFSH=global, LFmGLU=global, LFmHAM=global, LFmHFL=global, LFmRF=global, LFmVAS=global, LHipStop=global, LKneeStop=global, LLceBFSH=global, LLceGLU=global, LLceHAM=global, LLceHFL=global, LLceRF=global, LLceVAS=global, LLmtuBFSH=global, LLmtuGLU=global, LLmtuHAM=global, LLmtuHFL=global, LLmtuRF=global, LLmtuVAS=global, LM12=global, LM23=global, LVceBFSH=global, LVceGLU=global, LVceHAM=global, LVceHFL=global, LVceRF=global, LVceVAS=global, LrBFSH=global, LrGLU=global, LrHAMh=global, LrHAMk=global, LrHFL=global, LrRFh=global, LrRFk=global, LrVAS=global, RActBFSH=global, RActGLU=global, RActHAM=global, RActHFL=global, RActRF=global, RActVAS=global, RFmBFSH=global, RFmGLU=global, RFmHAM=global, RFmHFL=global, RFmRF=global, RFmVAS=global, RHipStop=global, RKneeStop=global, RLceBFSH=global, RLceGLU=global, RLceHAM=global, RLceHFL=global, RLceRF=global, RLceVAS=global, RLmtuBFSH=global, RLmtuGLU=global, RLmtuHAM=global, RLmtuHFL=global, RLmtuRF=global, RLmtuVAS=global, RM12=global, RM23=global, RVceBFSH=global, RVceGLU=global, RVceHAM=global, RVceHFL=global, RVceRF=global, RVceVAS=global, RrBFSH=global, RrGLU=global, RrHAMh=global, RrHAMk=global, RrHFL=global, RrRFh=global, RrRFk=global, RrVAS=global
  wires:
  [Lphi12] -> L Knee Joint Limits/1(phi [rad]1), VAS Link/1(phi23 [rad]), RF Link/2(phi23 [rad]), HAM Link/2(phi23 [rad]), L BFSH Link/1(phi23 [rad])
  [LStimHAM] -> HAM/1(STIM)
  HAM/1(Fmtc) -> Product9/1, Product8/1, [LFmHAM]
  HAM/2(Lce) -> R HAM Muscle Spindles1/1
  HFL/1(Fmtc) -> Product7/2, [LFmHFL]
  HFL/2(Lce) -> L HFL Muscle Spindles/1
  [LStimHFL] -> HFL/1(STIM)
  GLU/1(Fmtc) -> Product6/1, [LFmGLU]
  [LStimGLU] -> GLU/1(STIM)
  Sum16/1 -> [LM23]
  [Ldphi12] -> L Knee Joint Limits/2(dphi [rad/s]1)
  VAS Link/1(lmtu [m]) -> VAS/2(lmtc [m]), [LLmtuVAS]
  HAM Link/1(lmtu [m]) -> HAM/2(lmtc [m]), [LLmtuHAM]
  HAM Link/2(lever34 [m]) -> Product8/2, [LrHAMh]
  HAM Link/3(lever23 [m]) -> Product9/2, [LrHAMk]
  Sum3/1 -> Sum14/1
  [Lphi23] -> L Hip Joint Limits/1(phi [rad]1), HFL Link/1(phi34 [rad]), GLU Link/1(phi34 [rad]), RF Link/1(phi34 [rad]), HAM Link/1(phi34 [rad])
  VAS/4(A) -> [LActVAS]
  VAS/1(Fmtc) -> Product4/2, [LFmVAS]
  Sum1/1 -> [LM12]
  L Knee Joint Limits/1(M_stop [Nm]1) -> Sum1/1, [LKneeStop]
  Sum5/1 -> Sum1/2
  VAS Link/2(lever [m]) -> [LrVAS], Product4/1
  Sum22/1 -> Sum5/1
  HAM/4(A) -> [LActHAM]
  Product8/1 -> Sum3/2
  Product6/1 -> Sum3/1
  GLU Link/1(lmtu [m]) -> GLU/2(lmtc [m]), [LLmtuGLU]
  GLU Link/2(lever [m]) -> Product6/2, [LrGLU]
  GLU/4(A) -> [LActGLU]
  [Ldphi23] -> L Hip Joint Limits/2(dphi [rad/s]1)
  L Hip Joint Limits/1(M_stop [Nm]1) -> [LHipStop], Sum16/1
  Sum14/1 -> Sum16/2
  HFL Link/1(lmtu [m]) -> HFL/2(lmtc [m]), [LLmtuHFL]
  HFL/4(A) -> [LActHFL]
  HFL Link/2(lever [m]) -> Product7/1, [LrHFL]
  [LStimVAS] -> VAS/1(STIM)
  GLU/2(Lce) -> L HFL Muscle Spindles3/1
  GLU/3(Vce) -> L HFL Muscle Spindles2/1
  HAM/3(Vce) -> R HAM Muscle Spindles6/1
  VAS/3(Vce) -> L RF Muscle Spindles6/1
  VAS/2(Lce) -> L RF Muscle Spindles4/1
  HFL/3(Vce) -> L HFL Muscle Spindles1/1
  RF/4(A) -> [LActRF]
  RF/3(Vce) -> L RF Muscle Spindles2/1
  RF/2(Lce) -> L RF Muscle Spindles/1
  RF Link/1(lmtu [m]) -> [LLmtuRF], RF/2(lmtc [m])
  RF Link/2(lever34 [m]) -> Product5/1, [LrRFh]
  RF Link/3(lever23 [m]) -> Product15/1, [LrRFk]
  [LStimRF] -> RF/1(STIM)
  Product7/1 -> Sum11/1
  Product5/1 -> Sum11/2
  Product15/1 -> Sum17/2
  Sum17/1 -> Sum5/2
  Product4/1 -> Sum17/1
  [LStimBFSH] -> BFSH/1(STIM)
  L BFSH Link/1(lmtu [m]) -> BFSH/2(lmtc [m]), [LLmtuBFSH]
  L BFSH Link/2(lever [m]) -> [LrBFSH], Product20/2
  BFSH/4(A) -> [LActBFSH]
  BFSH/2(Lce) -> R HAM Muscle Spindles4/1
  BFSH/3(Vce) -> R HAM Muscle Spindles2/1
  Product20/1 -> Sum22/2
  Product9/1 -> Sum22/1
  L HFL Muscle Spindles1/1 -> [LVceHFL]
  L HFL Muscle Spindles2/1 -> [LVceGLU]
  L HFL Muscle Spindles3/1 -> [LLceGLU]
  L RF Muscle Spindles6/1 -> [LVceVAS]
  RF/1(Fmtc) -> Product5/2, Product15/2, [LFmRF]
  BFSH/1(Fmtc) -> Product20/1, [LFmBFSH]
  L HFL Muscle Spindles/1 -> [LLceHFL]
  R HAM Muscle Spindles1/1 -> [LLceHAM]
  R HAM Muscle Spindles6/1 -> [LVceHAM]
  L RF Muscle Spindles/1 -> [LLceRF]
  L RF Muscle Spindles2/1 -> [LVceRF]
  R HAM Muscle Spindles4/1 -> [LLceBFSH]
  R HAM Muscle Spindles2/1 -> [LVceBFSH]
  L RF Muscle Spindles4/1 -> [LLceVAS]
  [Rphi12] -> L Knee Joint Limits1/1(phi [rad]1), VAS Link1/1(phi23 [rad]), HAM Link1/2(phi23 [rad]), RF Link1/2(phi23 [rad]), L BFSH Link1/1(phi23 [rad])
  [RStimHAM] -> HAM1/1(STIM)
  HAM1/1(Fmtc) -> Product23/1, Product22/1, [RFmHAM]
  HAM1/2(Lce) -> R HAM Muscle Spindles3/1
  HFL1/1(Fmtc) -> Product21/2, [RFmHFL]
  HFL1/2(Lce) -> L HFL Muscle Spindles4/1
  [RStimHFL] -> HFL1/1(STIM)
  GLU1/1(Fmtc) -> Product19/1, [RFmGLU]
  [RStimGLU] -> GLU1/1(STIM)
  Sum12/1 -> [RM23]
  [Rdphi12] -> L Knee Joint Limits1/2(dphi [rad/s]1)
  VAS Link1/1(lmtu [m]) -> VAS1/2(lmtc [m]), [RLmtuVAS]
  HAM Link1/1(lmtu [m]) -> HAM1/2(lmtc [m]), [RLmtuHAM]
  HAM Link1/2(lever34 [m]) -> Product22/2, [RrHAMh]
  HAM Link1/3(lever23 [m]) -> Product23/2, [RrHAMk]
  Sum19/1 -> Sum10/1
  [Rphi23] -> L Hip Joint Limits1/1(phi [rad]1), HFL Link1/1(phi34 [rad]), GLU Link1/1(phi34 [rad]), RF Link1/1(phi34 [rad]), HAM Link1/1(phi34 [rad])
  VAS1/4(A) -> [RActVAS]
  VAS1/1(Fmtc) -> Product17/2, [RFmVAS]
  Sum7/1 -> [RM12]
  L Knee Joint Limits1/1(M_stop [Nm]1) -> Sum7/1, [RKneeStop]
  Sum21/1 -> Sum7/2
  VAS Link1/2(lever [m]) -> [RrVAS], Product17/1
  Sum18/1 -> Sum21/1
  HAM1/4(A) -> [RActHAM]
  Product22/1 -> Sum19/2
  Product19/1 -> Sum19/1
  GLU Link1/1(lmtu [m]) -> GLU1/2(lmtc [m]), [RLmtuGLU]
  GLU Link1/2(lever [m]) -> Product19/2, [RrGLU]
  GLU1/4(A) -> [RActGLU]
  [Rdphi23] -> L Hip Joint Limits1/2(dphi [rad/s]1)
  L Hip Joint Limits1/1(M_stop [Nm]1) -> [RHipStop], Sum12/1
  Sum10/1 -> Sum12/2
  HFL Link1/1(lmtu [m]) -> [RLmtuHFL], HFL1/2(lmtc [m])
  HFL1/4(A) -> [RActHFL]
  HFL Link1/2(lever [m]) -> Product21/1, [RrHFL]
  [RStimVAS] -> VAS1/1(STIM)
  GLU1/2(Lce) -> L HFL Muscle Spindles7/1
  GLU1/3(Vce) -> L HFL Muscle Spindles6/1
  HAM1/3(Vce) -> R HAM Muscle Spindles14/1
  VAS1/3(Vce) -> L RF Muscle Spindles7/1
  VAS1/2(Lce) -> L RF Muscle Spindles5/1
  HFL1/3(Vce) -> L HFL Muscle Spindles5/1
  RF1/4(A) -> [RActRF]
  RF1/3(Vce) -> L RF Muscle Spindles3/1
  RF1/2(Lce) -> L RF Muscle Spindles1/1
  RF Link1/1(lmtu [m]) -> RF1/2(lmtc [m]), [RLmtuRF]
  RF Link1/2(lever34 [m]) -> Product18/1, [RrRFh]
  RF Link1/3(lever23 [m]) -> [RrRFk], Product12/1
  [RStimRF] -> RF1/1(STIM)
  Sum8/1 -> Sum10/2
  Product21/1 -> Sum8/1
  Product18/1 -> Sum8/2
  Product12/1 -> Sum13/2
  Sum13/1 -> Sum21/2
  Product17/1 -> Sum13/1
  [RStimBFSH] -> BFSH1/1(STIM)
  L BFSH Link1/1(lmtu [m]) -> BFSH1/2(lmtc [m]), [RLmtuBFSH]
  L BFSH Link1/2(lever [m]) -> [RrBFSH], Product14/2
  BFSH1/4(A) -> [RActBFSH]
  BFSH1/2(Lce) -> R HAM Muscle Spindles13/1
  BFSH1/3(Vce) -> R HAM Muscle Spindles12/1
  Product14/1 -> Sum18/2
  Product23/1 -> Sum18/1
  L HFL Muscle Spindles5/1 -> [RVceHFL]
  L HFL Muscle Spindles6/1 -> [RVceGLU]
  L HFL Muscle Spindles7/1 -> [RLceGLU]
  L RF Muscle Spindles7/1 -> [RVceVAS]
  RF1/1(Fmtc) -> Product18/2, Product12/2, [RFmRF]
  BFSH1/1(Fmtc) -> Product14/1, [RFmBFSH]
  L HFL Muscle Spindles4/1 -> [RLceHFL]
  R HAM Muscle Spindles3/1 -> [RLceHAM]
  R HAM Muscle Spindles14/1 -> [RVceHAM]
  L RF Muscle Spindles1/1 -> [RLceRF]
  L RF Muscle Spindles3/1 -> [RVceRF]
  R HAM Muscle Spindles13/1 -> [RLceBFSH]
  R HAM Muscle Spindles12/1 -> [RVceBFSH]
  L RF Muscle Spindles5/1 -> [RLceVAS]
  Sum11/1 -> Sum14/2

== system atrias_boom_nmSt_kinSw_v3/Control/Behavior Control/Virtual Neuromuscular Control/Neural Control Layer ==
  note: Neural Control Layer
      | (Sagittal Plane)
  Constant1 : Constant  Value=zeros(4,1)  OutDataTypeStr=boolean
  Constant18 : Constant  OutDataTypeStr=boolean
  Constant2 : Constant  Value=zeros(4,1)  OutDataTypeStr=boolean
  Constant3 : Constant  OutDataTypeStr=boolean
  Demux1 : Demux  Outputs=6
  Demux3 : Demux  Outputs=6
  L Stance Phase (sagittal) : Subsystem  TreatAsAtomicUnit=on
  "L Stance, Swing, Trans (sagittal)" : Subsystem
  MDelay{1..4} (4 alike) : Delay  DelayLength=MidDelay_discrete  InitialCondition=0  SampleTime=sample_time
  Mux1 : Mux  Inputs=2
  Mux2 : Mux  Inputs=2
  R Stance Phase (sagittal) : Subsystem  TreatAsAtomicUnit=on
  "R Stance, Swing, Trans (sagittal)" : Subsystem
  Saturation1 : Saturate  UpperLimit=1  LowerLimit=0.01  ZeroCross=off
  Saturation10 : Saturate  UpperLimit=1  LowerLimit=0.01  ZeroCross=off
  tag scope: LAct=global, LStance=global, LStimBFSH=global, LStimGLU=global, LStimHAM=global, LStimHFL=global, LStimRF=global, LStimVAS=global, LSwingPhase=global, RAct=global, RStance=global, RStimBFSH=global, RStimGLU=global, RStimHAM=global, RStimHFL=global, RStimRF=global, RStimVAS=global, RSwingPhase=global
  wires:
  [StCtrlPar] -> L Stance Phase (sagittal)/1(CtrlPar)
  [LFmVAS] -> MDelay2/1
  MDelay2/1 -> MDelay3/1
  [LLceBFSH] -> L Stance Phase (sagittal)/5(LceBFSH)
  Constant18/1 -> L Stance Phase (sagittal)/Enable, [LStance]
  Saturation10/1 -> Demux3/1
  Demux3/1 -> [LStimHFL]  "HFL"
  Demux3/2 -> [LStimGLU]  "GLU"
  Demux3/3 -> [LStimHAM]  "HAM"
  Demux3/4 -> [LStimRF]  "RF"
  Demux3/5 -> [LStimVAS]  "VAS"
  Demux3/6 -> [LStimBFSH]  "BFSH"
  L Stance Phase (sagittal)/1(S_St_0) -> "L Stance, Swing, Trans (sagittal)"/2(S_0_St)
  L Stance Phase (sagittal)/2(S_M1 [VAS]) -> "L Stance, Swing, Trans (sagittal)"/3(S_M1)
  L Stance Phase (sagittal)/3(S_M2 [VAS BFSH]) -> "L Stance, Swing, Trans (sagittal)"/4(S_M2)
  [theta] -> Mux2/1
  [dtheta] -> Mux2/2
  [theta_tgt] -> L Stance Phase (sagittal)/2(theta_tgt [rad])
  [LLLoad] -> "L Stance, Swing, Trans (sagittal)"/1(ILLoad)
  L Stance Phase (sagittal)/4(S_M3 [HFL GLU HAM]) -> "L Stance, Swing, Trans (sagittal)"/5(S_M3)
  Mux2/1 -> L Stance Phase (sagittal)/3(theta dtheta [rad rad/s])
  "L Stance, Swing, Trans (sagittal)"/2(S_Modules) -> [LAct]
  MDelay3/1 -> L Stance Phase (sagittal)/4(FmVAS)
  Constant1/1 -> [LSwingPhase]
  [StCtrlPar] -> R Stance Phase (sagittal)/1(CtrlPar)
  [RFmVAS] -> MDelay1/1
  MDelay1/1 -> MDelay4/1
  [RLceBFSH] -> R Stance Phase (sagittal)/5(LceBFSH)
  Constant3/1 -> R Stance Phase (sagittal)/Enable, [RStance]
  Saturation1/1 -> Demux1/1
  Demux1/1 -> [RStimHFL]  "HFL"
  Demux1/2 -> [RStimGLU]  "GLU"
  Demux1/3 -> [RStimHAM]  "HAM"
  Demux1/4 -> [RStimRF]  "RF"
  Demux1/5 -> [RStimVAS]  "VAS"
  Demux1/6 -> [RStimBFSH]  "BFSH"
  R Stance Phase (sagittal)/1(S_St_0) -> "R Stance, Swing, Trans (sagittal)"/2(S_0_St)
  R Stance Phase (sagittal)/2(S_M1 [VAS]) -> "R Stance, Swing, Trans (sagittal)"/3(S_M1)
  R Stance Phase (sagittal)/3(S_M2 [VAS BFSH]) -> "R Stance, Swing, Trans (sagittal)"/4(S_M2)
  [theta] -> Mux1/1
  [dtheta] -> Mux1/2
  [theta_tgt] -> R Stance Phase (sagittal)/2(theta_tgt [rad])
  [RLLoad] -> "R Stance, Swing, Trans (sagittal)"/1(ILLoad)
  R Stance Phase (sagittal)/4(S_M3 [HFL GLU HAM]) -> "R Stance, Swing, Trans (sagittal)"/5(S_M3)
  Mux1/1 -> R Stance Phase (sagittal)/3(theta dtheta [rad rad/s])
  "R Stance, Swing, Trans (sagittal)"/2(S_Modules) -> [RAct]
  MDelay4/1 -> R Stance Phase (sagittal)/4(FmVAS)
  Constant2/1 -> [RSwingPhase]
  "L Stance, Swing, Trans (sagittal)"/1(S) -> Saturation10/1
  "R Stance, Swing, Trans (sagittal)"/1(S) -> Saturation1/1

== system atrias_boom_nmSt_kinSw_v3/Control/Behavior Control/Virtual Neuromuscular Control/Torque Distribution ==
  note: J^(-T) [tauB; tauF] = [tauH, tauK]
  note: Map Torques
  note: J^(-T) [tauB; tauF] = [tauH, tauK]
  R tauK_des [Nm] : Inport
  R tauH_des [Nm] : Inport  Port=2
  R Jacobian Constant (k) : Inport  Port=3
  L tauK_des [Nm] : Inport  Port=4
  L tauH_des [Nm] : Inport  Port=5
  L Jacobian Constant (k) : Inport  Port=6
  Demux : Demux
  Demux1 : Demux  Outputs=2
  Demux2 : Demux  Outputs=2
  Mux : Mux
  Mux1 : Mux  Inputs=2
  Mux2 : Mux  Inputs=2
  Switch1 : Switch  Criteria=u2 > Threshold
  Switch2 : Switch  Criteria=u2 > Threshold
  Torque Limiter (outside) 1 : Saturate  UpperLimit=max_sagittal_loaded_torque  LowerLimit=-max_sagittal_loaded_torque
      settings: AttributesFormatString=Hi: %<UpperLimit>\nLo: %<LowerLimit>
  Torque Limiter (outside) 2 : Saturate  UpperLimit=max_sagittal_loaded_torque  LowerLimit=-max_sagittal_loaded_torque
      settings: AttributesFormatString=Hi: %<UpperLimit>\nLo: %<LowerLimit>
  Torque Limiter (outside) 3 : Saturate  UpperLimit=max_sagittal_unloaded_torque  LowerLimit=-max_sagittal_unloaded_torque
      settings: AttributesFormatString=Hi: %<UpperLimit>\nLo: %<LowerLimit>
  Torque Limiter (outside) 4 : Saturate  UpperLimit=max_sagittal_unloaded_torque  LowerLimit=-max_sagittal_unloaded_torque
      settings: AttributesFormatString=Hi: %<UpperLimit>\nLo: %<LowerLimit>
  map_tau_L : MATLAB Function  TreatAsAtomicUnit=on
  map_tau_R : MATLAB Function  TreatAsAtomicUnit=on
  mech limit avoidance1 : Subsystem  Commented=on
  R tauB [Nm] : Outport
  R tauF [Nm] : Outport  Port=2
  R J_inv_transpose [2x2] : Outport  Port=3
  L tauB [Nm] : Outport  Port=4
  L tauF [Nm] : Outport  Port=5
  L J_inv_transpose [2x2] : Outport  Port=6
  wires:
  R Jacobian Constant (k)/1 -> map_tau_R/3(k)
  map_tau_R/3(Jinv_trans) -> R J_inv_transpose [2x2]/1
  L Jacobian Constant (k)/1 -> map_tau_L/3(k)
  map_tau_L/3(Jinv_trans) -> L J_inv_transpose [2x2]/1
  map_tau_L/1(tauB) -> Mux2/1
  map_tau_L/2(tauF) -> Mux2/2
  Mux/1 -> Demux/1
  Demux/1 -> [RtauH]
  R tauH_des [Nm]/1 -> Mux/1
  R tauK_des [Nm]/1 -> Mux/2
  L tauH_des [Nm]/1 -> Mux/3
  L tauK_des [Nm]/1 -> Mux/4
  Demux/2 -> [RtauK]
  Demux/3 -> [LtauH]
  Demux/4 -> [LtauK]
  [RtauH] -> map_tau_R/1(tauH_des)
  [RtauK] -> map_tau_R/2(tauK_des)
  [LtauH] -> map_tau_L/1(tauH_des)
  [LtauK] -> map_tau_L/2(tauK_des)
  Switch1/1 -> Demux1/1
  [LFootCnt] -> Switch1/2
  Mux2/1 -> Torque Limiter (outside) 1/1, Torque Limiter (outside) 3/1
  Torque Limiter (outside) 3/1 -> Switch1/3
  Torque Limiter (outside) 1/1 -> Switch1/1
  Demux1/2 -> L tauF [Nm]/1
  Demux1/1 -> L tauB [Nm]/1
  map_tau_R/1(tauB) -> Mux1/1
  map_tau_R/2(tauF) -> Mux1/2
  Switch2/1 -> Demux2/1
  [RFootCnt] -> Switch2/2
  Mux1/1 -> Torque Limiter (outside) 2/1, Torque Limiter (outside) 4/1
  Torque Limiter (outside) 4/1 -> Switch2/3
  Torque Limiter (outside) 2/1 -> Switch2/1
  Demux2/2 -> R tauF [Nm]/1
  Demux2/1 -> R tauB [Nm]/1

== system atrias_boom_nmSt_kinSw_v3/Control/Behavior Control/command routing/(M4) Swing Leg Complensation ==
  RTorques : Inport
  LTorques : Inport  Port=2
  RLeg in Sw [1/0] : Inport  Port=3
  LLeg in Sw [1/0] : Inport  Port=4
  M4_G : Inport  Port=5
  Demux1 : Demux  Outputs=2
  Logical Operator : Logic  Operator=OR  AllPortsSameDT=off  OutDataTypeStr=boolean
  Logical Operator1 : Logic  Operator=NOT  AllPortsSameDT=off  OutDataTypeStr=boolean
  Logical Operator2 : Logic  Operator=NOT  AllPortsSameDT=off  OutDataTypeStr=boolean
  Mux1 : Mux  Inputs=2
  Mux2 : Mux  Inputs=2
  Swing Leg Compensation : Subsystem
  Switch{,1..4} (5 alike) : Switch  Criteria=u2 ~= 0
  RTorques_comp : Outport
  LTorques_comp : Outport  Port=2
  wires:
  [LLegInSw] -> Logical Operator1/1, Switch1/2, Logical Operator/2
  [RLegInSw] -> Logical Operator/1
  Logical Operator/1 -> Switch/2
  [LTorques] -> Mux1/2, Switch2/3, Switch1/3
  [RTorques] -> Switch2/1, Switch1/1, Mux1/1
  Switch1/1 -> Swing Leg Compensation/1(StTorques)
  Logical Operator1/1 -> Switch2/2
  Switch2/1 -> Swing Leg Compensation/2(SwTorques)
  Swing Leg Compensation/1(StTorques_comp) -> Switch4/1, Switch3/1  "St"
  Swing Leg Compensation/2(SwTorques_comp) -> Switch3/3, Switch4/3  "Sw"
  RTorques/1 -> [RTorques]
  LTorques/1 -> [LTorques]
  RLeg in Sw [1/0]/1 -> [RLegInSw]
  LLeg in Sw [1/0]/1 -> [LLegInSw]
  [LLegInSw] -> Logical Operator2/1, Switch3/2
  Logical Operator2/1 -> Switch4/2
  Switch3/1 -> Mux2/1
  Switch4/1 -> Mux2/2
  Mux2/1 -> Switch/1
  Mux1/1 -> Switch/3
  Switch/1 -> Demux1/1
  Demux1/1 -> RTorques_comp/1
  Demux1/2 -> LTorques_comp/1
  M4_G/1 -> [M4_G]
  [M4_G] -> Swing Leg Compensation/3(M4_G)

== system atrias_boom_nmSt_kinSw_v3/Control/Behavior Control/command routing/Desired Torque Derivative (left) ==
  x : Inport
  flight [1/0] : Inport  Port=2
  Detect Change : simulink/Logic and Bit Operations/Detect Change  vinit=0  InputProcessing=Inherited  OutDataTypeStr=boolean
  Gain1 : Gain  Gain=1/sample_time
  Logical Operator : Logic  Operator=NOT  AllPortsSameDT=off  OutDataTypeStr=boolean
  Product : Product
  difference : simulink/Discrete/Difference  ICPrevInput=0.0  InputProcessing=Inherited  OutMin=[]  OutMax=[]  OutDataType=fixdt(1, 16)  OutScaling=2^-10  DoSatur=off
  two_pole_filter : DiscreteTransferFcn  Numerator=[A_lpf_dtau 0 0]  Denominator=[1 B1_lpf_dtau B2_lpf_dtau]  ExternalReset=Either  SampleTime=sample_time
      settings: InputPortMap=u0,r7
  dx/dt : Outport
  wires:
  Logical Operator/1 -> Product/2
  Detect Change/1 -> Logical Operator/1
  Product/1 -> two_pole_filter/1
  difference/1 -> Product/1
  flight [1/0]/1 -> Detect Change/1, two_pole_filter/2
  two_pole_filter/1 -> dx/dt/1
  x/1 -> Gain1/1
  Gain1/1 -> difference/1
